simulink model "Cruise_control"  (R2020a)
settings: Solver=ode45  StartTime=0.0  StopTime=120  RelTol=1e-3
values from neighbouring files (symbols this model uses):
  b = 50.0    [data.sldd]
  m = 1000.0    [data.sldd]
undefined symbols (not defined in the file or in its folder): Ki, Kp, Ts
settings Model: DataDictionary=data.sldd  Creator=kolep  LastModifiedBy=kolep

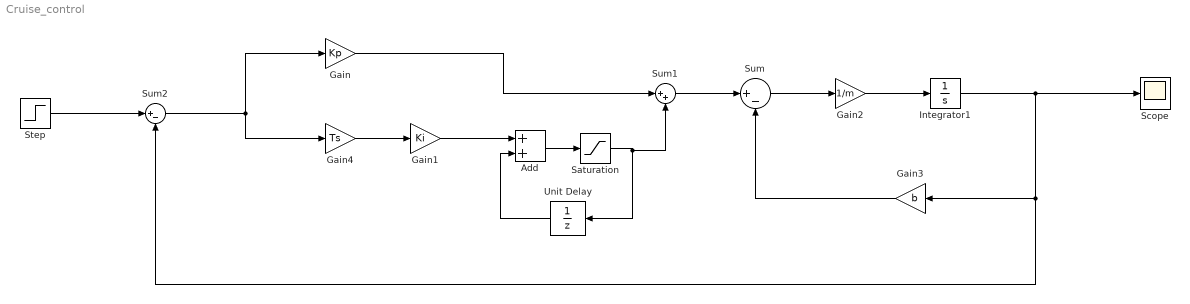
== system Cruise_control ==
  Add : Sum
  Gain : Gain  Gain=Kp
  Gain1 : Gain  Gain=Ki
  Gain2 : Gain  Gain=1/m
  Gain3 : Gain  Gain=b
  Gain4 : Gain  Gain=Ts
  Integrator1 : Integrator
  Saturation : Saturate
  Scope : Scope
  Step : Step  After=u  SampleTime=0
  Sum : Sum  Inputs=|+-
  Sum1 : Sum  Inputs=|++
  Sum2 : Sum  Inputs=|+-
  Unit Delay : UnitDelay  SampleTime=-1  HasFrameUpgradeWarning=on
  wires:
  Saturation/1 -> Sum1/2, Unit Delay/1
  Sum/1 -> Gain2/1
  Integrator1/1 -> Gain3/1, Sum2/2, Scope/1
  Gain2/1 -> Integrator1/1
  Gain3/1 -> Sum/2
  Add/1 -> Saturation/1
  Gain4/1 -> Gain1/1
  Gain/1 -> Sum1/1
  Sum1/1 -> Sum/1
  Gain1/1 -> Add/1
  Unit Delay/1 -> Add/2
  Step/1 -> Sum2/1
  Sum2/1 -> Gain4/1, Gain/1
